simulink model "VCU_SW_2020"  (R2020b)
settings: Solver=FixedStepDiscrete  StartTime=0.0  StopTime=inf  FixedStep=1e-2  RelTol=1e-3
PreLoadFcn:
  | RTWConfigurationCB('preloadfcn', bdroot);
InitFcn:
  | loadvar_ttc500
undefined symbols (not defined in the file): BrkPedalTypes, CabMovModeTypes, cFuseTempSensAcc_X, cFuseTempSensAcc_Y, cFuseTempSensVal_X, cFuseTempSensVal_Y, cTMSTempSensVal_X, cTMSTempSensVal_Y, cTransferCaseSpeedRatio, diag_state, DoorsPositionTypes, dP_filter_Y, DriverOccClassSystemTypes, ErrorValueTypes, fatal_error_callback, IO_ADC_NO_RANGE, LadderStatusTypes, pAnalogCabRotSensAcc, pAnalogCabRotSensMaxVolt, pAnalogCabRotSensMinVolt, pAnalogCabRotSensRange, pAnalogCabRotSensZeroVolt, pBrkActivePress, pCabTiltSensAcc, pCabTiltSensMaxCur, pCabTiltSensMinCur, pDistanceCorrection, pECANManual_BPNEnable, pECANManual_BPNEnabler_Flag, pFilterSensAccRes, pHDirMaxDiffFrq, pHDirSensHighLvl, pHDirSensLowLvl, pMainGearRatio, pMaxFilterSensRes, pMaxFirstPedalSensValue, pMaxFuseTempSensRes, pMaxPressLoss, pMaxPressSensCurrent, pMaxPressValue, pMaxPressValueHydMotAndPump, pMaxPressValueParkDrain, pMaxSecondPedalSensValue, pMaxTempSensVoltage, pMaxTempValue, pMaxTMSTempSensRes, pMinFilterSensRes, pMinFirstPedalSensValue, pMinFuseTempSensRes, pMinPressLoss, pMinPressSensCurrent, pMinPressValue, pMinSecondPedalSensValue, pMinTempSensVoltage, pMinTempValue, pMinTMSTempSensRes, pMotorRingTeethNum, pPedalSensAccuracyPct, pPedalSensAccuracyVolt, pPressLossTreshhold ... (+20)
libraries: TTlibrary x270, canmsglib x127, simulink x88
(part 16 of 17)

== matlab function VCU_SW_2020/ServerFcn/convDIOStatusTypeToNum/MATLAB Function ==
  data: enum input; value output
function value = convertDIOStsToNumFcn(enum)
%#codegen
    if enum == StatusModeTypes.ON
        value = true;
    else
        value = false;
    end
% for future, if there is error or warning, then set function is not called
end

== matlab function VCU_SW_2020/InputLayer/InputInterfaces/AnalogInput/AIProc10msec/WasherTiltPumpTrans/getWasherTiltPumpTransSensDataFcn ==
  data: washerTiltPumpTransSens input; washerTiltPercent output; maxVolt input; minVolt input; accuracy input
function washerTiltPercent = getAnalogCabRotSensData(washerTiltPumpTransSens,...
     maxVolt, minVolt, accuracy)

 sensRange = single(maxVolt - minVolt)/single(2);
 zeroVolt = single(minVolt) + sensRange;
 
if (washerTiltPumpTransSens > (minVolt - accuracy)) &&...
   (washerTiltPumpTransSens < (maxVolt + accuracy)) %условие на попадание в диапазон датчика, при невыполнении - ошибка
    if washerTiltPumpTransSens > maxVolt %крайнее положение - остается
        washerTiltPercent = int8(100);
    elseif washerTiltPumpTransSens < minVolt %крайнее положение - остается
        washerTiltPercent = -int8(100);
    else
        if washerTiltPumpTransSens > zeroVolt
            helper = (single(washerTiltPumpTransSens) - single(zeroVolt))/single(sensRange)*single(100);
        elseif washerTiltPumpTransSens < zeroVolt 
            helper = -(single(zeroVolt) - single(washerTiltPumpTransSens))/single(sensRange)*single(100);
        else
            helper = single(0);
        end
        washerTiltPercent = int8(helper);
    end
else
   washerTiltPercent = int8(ErrorValueTypes.UNKNOWN_ERROR); 
end 
    
end

== matlab function VCU_SW_2020/InputLayer/InputInterfaces/DigitalInput/Function-Call Subsystem/MATLAB Function ==
  data: sensSupply1 input; sensSupply2 input
  events: fcncall output FUNCTION_CALL_EVENT
function fcn(sensSupply1, sensSupply2)

    persistent timer
        if isempty(timer)
            timer = uint8(0);
        end
        
    if sensSupply1 == StateModeTypes.STT_ENABLE && sensSupply2 == StateModeTypes.STT_ENABLE
        if timer < uint8(1000)
            timer = timer + uint8(1);
        end
    end
    
    if timer >= uint8(1000)
        fcncall();
    end
    
end

== matlab function VCU_SW_2020/InputLayer/InputInterfaces/DigitalInput/Function-Call Subsystem/cabRotIndSensProc/cabRotIndSensProc fcn ==
  data: pResetIndCabSensErr input
function cabRotIndSensProc(pResetIndCabSensErr)
    
    persistent err
    if isempty(err)
        err = false;
    end
    
    if err
        if pResetIndCabSensErr
            err = false;
            setIndSensErr(err);
        end        
    else
        cabRotPos = getIndRotSensData();
        if cabRotPos == CabRotPosTypes.ROTPOS_ERROR
            err = true;
            setIndSensErr(err);
        else
            setIndRotSensData(cabRotPos);
        end        
    end

end

== matlab function VCU_SW_2020/InputLayer/InputInterfaces/DigitalInput/Function-Call Subsystem/cabRotIndSensProc/getIndRotSensData/getIndRotSensData fcn ==
  data: indSensLeft input; cabPos output; indSensRight input
function cabPos = getIndRotSensData(indSensLeft, indSensRight)

    if (indSensRight == StateModeTypes.STT_ENABLE)&&...
       (indSensLeft == StateModeTypes.STT_ENABLE)
        cabPos = CabRotPosTypes.ROTPOS_NEAR_ZERO;
    elseif (indSensRight == StateModeTypes.STT_DISABLE)&&...
           (indSensLeft == StateModeTypes.STT_ENABLE)
        cabPos = CabRotPosTypes.ROTPOS_LEFT;
    elseif (indSensRight == StateModeTypes.STT_ENABLE)&&...
           (indSensLeft == StateModeTypes.STT_DISABLE)
        cabPos = CabRotPosTypes.ROTPOS_RIGHT;
    elseif (indSensRight == StateModeTypes.STT_DISABLE)&&...
           (indSensLeft == StateModeTypes.STT_DISABLE)
        switch getRotPos()
            case {CabRotPosTypes.ROTPOS_LEFT, CabRotPosTypes.ROTPOS_LEFT_END}
                cabPos = CabRotPosTypes.ROTPOS_LEFT_END;
            case {CabRotPosTypes.ROTPOS_RIGHT, CabRotPosTypes.ROTPOS_RIGHT_END}
                cabPos = CabRotPosTypes.ROTPOS_RIGHT_END;
            otherwise
                cabPos = CabRotPosTypes.ROTPOS_ERROR;
        end    
    else
        cabPos = CabRotPosTypes.ROTPOS_ERROR;
    end
    
end

== matlab function VCU_SW_2020/InputLayer/InputInterfaces/PWDInput/PWDProc100msec/MATLAB Function ==
  data: HMotorSpeed input; vehicleSpeed output; trCaseGear input; wheelRad input; finalDriveRatio input; lowRatio input; highRatio input; diagReplacement input; diagErrorValue input
function vehicleSpeed  = calculateVehicleSpeed(HMotorSpeed, trCaseGear,...
    wheelRad, finalDriveRatio, lowRatio, highRatio, ...
    diagReplacement, diagErrorValue)

if diagErrorValue ~= StateModeTypes.STT_ENABLE && ...
        diagReplacement ~= StateModeTypes.STT_ENABLE && ...
        HMotorSpeed ~= uint16(ErrorValueTypes.SPEED_ERROR_VALUE)
    if trCaseGear == GearNumTypes.GEAR_2_WHEEL_LOW || trCaseGear == GearNumTypes.GEAR_4_WHEEL_LOW
        vehicleSpeedRaw = single(HMotorSpeed)*wheelRad*60*2*pi/lowRatio/finalDriveRatio/1000;
        vehicleSpeed = uint8(vehicleSpeedRaw);
    elseif trCaseGear == GearNumTypes.GEAR_2_WHEEL_HIGH || trCaseGear == GearNumTypes.GEAR_4_WHEEL_HIGH
        vehicleSpeedRaw = single(HMotorSpeed)*wheelRad*60*2*pi/highRatio/finalDriveRatio/1000;
        vehicleSpeed = uint8(vehicleSpeedRaw);
   elseif trCaseGear == GearNumTypes.GEAR_NEUTRAL || trCaseGear == GearNumTypes.GEAR_NOT_AVAILABLE
        vehicleSpeed = uint8(0);    
    else
        vehicleSpeed = uint8(ErrorValueTypes.SPEED_ERROR_VALUE);
    end
else
    vehicleSpeed = uint8(ErrorValueTypes.SPEED_ERROR_VALUE);
end

== matlab function VCU_SW_2020/InputLayer/InputInterfaces/DigitalInput/Function-Call Subsystem1/MATLAB Function ==
  data: HighGear input; state output; LowGear input
function state = transCaseStt(HighGear, LowGear)

if HighGear == StateModeTypes.STT_DISABLE && LowGear == StateModeTypes.STT_DISABLE
    state = GearNumTypes.GEAR_NOT_AVAILABLE;
elseif ( HighGear == StateModeTypes.STT_ENABLE && ...
        LowGear == StateModeTypes.STT_DISABLE)
    state = GearNumTypes.GEAR_2_WHEEL_HIGH;
elseif ( HighGear == StateModeTypes.STT_DISABLE && ...
        LowGear == StateModeTypes.STT_ENABLE)
    state = GearNumTypes.GEAR_4_WHEEL_LOW;
else
    state = GearNumTypes.GEAR_ERROR;
end

end

== matlab function VCU_SW_2020/InputLayer/InputNetwork/InputCCAN/CCAN100msecProc1/InputTransSelect/calcLeverPos/MATLAB Function ==
  data: TransReqGear input; SelSig1 input; LeverPos output; SelSig2 input; SelSig3 input
function LeverPos = calculateLeverPosition(TransReqGear, SelSig1,...
    SelSig2, SelSig3)


if (TransReqGear == LeverPosTypes.NEUTRAL && SelSig1 == StateModeTypes.STT_ENABLE && ...
        SelSig2 ==StateModeTypes.STT_DISABLE && SelSig3 == StateModeTypes.STT_DISABLE)
    LeverPos = LeverPosTypes.NEUTRAL;
elseif (TransReqGear == LeverPosTypes.DRIVE && SelSig1 == StateModeTypes.STT_DISABLE && ...
        SelSig2 ==StateModeTypes.STT_ENABLE && SelSig3 == StateModeTypes.STT_DISABLE)
    LeverPos = LeverPosTypes.DRIVE;
elseif (TransReqGear == LeverPosTypes.REVERSE && SelSig1 == StateModeTypes.STT_DISABLE && ...
        SelSig2 ==StateModeTypes.STT_DISABLE && SelSig3 == StateModeTypes.STT_ENABLE)
    LeverPos = LeverPosTypes.REVERSE;
else
    if (SelSig1 == StateModeTypes.STT_ERROR || SelSig2 == StateModeTypes.STT_ERROR ||...
            SelSig3 == StateModeTypes.STT_ERROR)
        LeverPos = TransReqGear;
    elseif (TransReqGear == LeverPosTypes.LEVER_POS_ERROR || ...
            TransReqGear == LeverPosTypes.LEVER_POS_DOES_NOT_DEFINED)
        if (SelSig1 == StateModeTypes.STT_ENABLE && ...
                SelSig2 ==StateModeTypes.STT_DISABLE && SelSig3 == StateModeTypes.STT_DISABLE)
            LeverPos = LeverPosTypes.NEUTRAL;
        elseif (SelSig1 == StateModeTypes.STT_DISABLE && ...
                SelSig2 ==StateModeTypes.STT_ENABLE && SelSig3 == StateModeTypes.STT_DISABLE)
            LeverPos = LeverPosTypes.DRIVE;
        elseif (SelSig1 == StateModeTypes.STT_DISABLE && ...
                SelSig2 ==StateModeTypes.STT_DISABLE && SelSig3 == StateModeTypes.STT_ENABLE)
            LeverPos = LeverPosTypes.REVERSE;
        else
            LeverPos = LeverPosTypes.LEVER_POS_DOES_NOT_DEFINED;
        end
    else
        LeverPos = LeverPosTypes.LEVER_POS_DOES_NOT_DEFINED;
    end
end

== matlab function VCU_SW_2020/EEPROM Layer/calculate trip distance/calcTotalDistCtrl ==
  data: EEPROMData data_store_memory
  events: calcTotalDist output FUNCTION_CALL_EVENT
function calcTotalDistCtrl()
global EEPROMData

  if  EEPROMData.writingInProcessFl ~= StateModeTypes.STT_ENABLE
      calcTotalDist();
  end

end

== matlab function VCU_SW_2020/EEPROM Layer/calculate trip distance/EEPROM read1/calcTotalDist ==
  data: tripDist input; updDistM output; savedDistM input; savedDistKM input; savedDistKKM input; updDistKM output; updDistKKM output; updDistTotal output
function [updDistM, updDistKM, updDistKKM, updDistTotal] = calcTotalDist(tripDist, ...
    savedDistM, savedDistKM, savedDistKKM)

updDistTotal = tripDist ...
    + uint32(savedDistKKM) * uint32(1000000) ...
    + uint32(savedDistKM) * uint32(1000) ...
    + uint32(savedDistM);

if uint16((updDistTotal - uint32(500000)) / uint32(1000000)) < uint16(1000)
    updDistKKM = uint16((updDistTotal - uint32(500000)) / uint32(1000000));
else
   updDistKKM = uint16(0);
end

updDistKM = uint16((uint32(updDistTotal - uint32(updDistKKM) ...
    * uint32(1000000)) - uint32(500)) / uint32(1000));

updDistM = uint16(updDistTotal - uint32(updDistKKM) * ...
    uint32(1000000) - uint32(updDistKM) * uint32(1000));

end

== matlab function VCU_SW_2020/EEPROM Layer/updateUDSStruct/MATLAB Function ==
  data: EngineHours input; UDSStruct data_store_memory
function fcn(EngineHours)

    global UDSStruct
    
    persistent EngineHoursOnStartup
        if isempty(EngineHoursOnStartup)
            EngineHoursOnStartup = single(UDSStruct.TotalEngineHours)*single(20);
        end
        
    UDSStruct.TotalEngineHours = uint32(EngineHoursOnStartup + EngineHours*single(20));
    UDSStruct.CurEngineHours = uint32(EngineHours*single(20));
    
end

== matlab function VCU_SW_2020/EEPROM Layer/Simulink Function/eeprom_read_processing_kora ==
  data: UDSStruct data_store_memory; flag output; read_sts output
function [flag, read_sts] = readProcessing()

    global UDSStruct
    
    %Флаг успешной записи в структуру
    flag = false;
    
    eeprom_read_sts = uint16(15);
    
    if (coder.target('MATLAB')) || (coder.target('Sfun'))

    else
        %Получение флага успешного чтения из EEPROM
        read_flag = uint8(0);
        read_flag = coder.ceval('get_read_flag');
        
        %Получение даных после второго успешного чтения
        %Первое успешное чтение обман (с) Ваня
        if read_flag == 2

            data = zeros(10, 1, 'uint32');
            coder.ceval('get_EEPROM_data', data);
            eeprom_read_sts = coder.ceval('get_readSts');

            UDSStruct.DistanceM = uint16(data(1));
            UDSStruct.DistanceKM = uint16(data(2));
            UDSStruct.DistanceKKM = uint16(data(3));
            UDSStruct.EngineHours = uint32(data(4));
            UDSStruct.TransPumpVolumeMax = uint8(data(5));
            UDSStruct.TransMotorVolumeMin = uint8(data(6));
            UDSStruct.AccelerationPedalMaxEngSpd = uint8(data(7));
            UDSStruct.AccelerationPedalMinEngSpd = uint8(data(8));
            UDSStruct.EngineSpeedMax = uint16(data(9));
            UDSStruct.EngineSpeedMin = uint16(data(10));
            
            flag = true;
            
        end
        
    end
    
    read_sts = eeprom_read_sts;
    
end

== matlab function VCU_SW_2020/EEPROM Layer/EEPROM Client2 ==
  data: t15common input; sig1 input; sig2 input; read_flag output; write_flag output
function [read_flag, write_flag] = EEPROMControl(t15common, sig1, sig2)
    
    persistent data_read_successful data_write_successful t15common_old read_reqest write_reqest
        if isempty(data_read_successful)
            data_read_successful = false;
            data_write_successful = false;
            t15common_old = StateModeTypes.STT_DISABLE;
            read_reqest = false;
            write_reqest = false;
        end
        
    persistent sig1_old sig2_old
        if isempty(sig1_old)
            sig1_old = StateModeTypes.STT_DISABLE;
            sig2_old = StateModeTypes.STT_DISABLE;
        end
        
    if t15common_old == StateModeTypes.STT_DISABLE ...
       && t15common == StateModeTypes.STT_ENABLE
        read_reqest = true;
    elseif t15common_old == StateModeTypes.STT_ENABLE ...
           && t15common == StateModeTypes.STT_DISABLE 
        write_reqest = true;
        setDataToWrite();
    end
        
    if ~data_read_successful && read_reqest == true ...
       || sig1 == StateModeTypes.STT_ENABLE ...
          && sig1_old == StateModeTypes.STT_DISABLE
        data_read_successful = readProcessing();
    end
    
    if ~data_write_successful && write_reqest == true ...
       || sig2 == StateModeTypes.STT_ENABLE ...
          && sig2_old == StateModeTypes.STT_DISABLE
        data_write_successful = writeProcessing();
    end
    
    sig1_old = sig1;
    sig2_old = sig2;
    
    t15common_old = t15common;
    
    read_flag = data_read_successful;
    write_flag = data_write_successful;
    
    get_eeprom_status();
        
end
% global EEPROMData
% persistent cnt exT15state rst_cnt
% if isempty(cnt)
%     cnt = uint8(0);
%     exT15state = t15common;
%     rst_cnt = uint8(0);
% end
% 
% if EEPROMData.alreadyReadFlag ~= StateModeTypes.STT_ENABLE
%     readDistance();
% end
% 
% if t15common ~= StateModeTypes.STT_ENABLE && exT15state == StateModeTypes.STT_ENABLE
%     EEPROMData.writingInProcessFl = StateModeTypes.STT_ENABLE;
% end
% 
% if EEPROMData.writingInProcessFl == StateModeTypes.STT_ENABLE && cnt < uint8(50)
%     cnt = cnt + uint8(1);
% else
%     EEPROMData.writingInProcessFl = StateModeTypes.STT_DISABLE;
%     if cnt ~= uint8(0)
%         cnt = uint8(0);
%     end
% end
% 
% if EEPROMData.writingInProcessFl == StateModeTypes.STT_ENABLE
%     if cnt == uint8(15)
%         if EEPROMData.updatedDistM ~= EEPROMData.savedDistM
%             write();
%         end
%     end
% 
%     if cnt == uint8(48)
%          EEPROMData.tripDistM = uint32(0);
%     end
% end
% 
% if tripReset == uint8(1)
%     
%     if rst_cnt < uint8(200)
%         
%         rst_cnt = rst_cnt + uint8(1);
%         
%     else
%        
%         if EEPROMData.Trip_Reset ~= StateModeTypes.STT_ENABLE
%             
%             EEPROMData.Trip_Reset = StateModeTypes.STT_ENABLE;
%             
%         end
%         
%     end
%     
% else
%     
%     if rst_cnt > uint8(0)
%         
%         rst_cnt = uint8(0);
%         
%     end
%     
%     if EEPROMData.Trip_Reset ~= StateModeTypes.STT_DISABLE
%         
%         EEPROMData.Trip_Reset = StateModeTypes.STT_DISABLE;
%         
%     end
%     
% end
% 
% exT15state = t15common;

== matlab function VCU_SW_2020/InputLayer/InputInterfaces/PWDInput/PWDProc100msec/validatePedalSensValue/MATLAB Function ==
  data: firstSensValue input; SpdValue output; secondSensValue input
function SpdValue = validateSpdSensValues(firstSensValue, ...
    secondSensValue)
    if and(firstSensValue ~= uint16(ErrorValueTypes.SPEED_ERROR_VALUE), ...
            secondSensValue ~= uint16(ErrorValueTypes.SPEED_ERROR_VALUE))
            helper = (uint16(firstSensValue) + ...
                uint16(secondSensValue))/uint16(2);
            SpdValue = uint16(helper);
    else
        SpdValue = uint16(ErrorValueTypes.SPEED_ERROR_VALUE);
    end
end

== matlab function VCU_SW_2020/InputLayer/InputInterfaces/AnalogInput/AIProc1000msec/Filter/MATLAB Function1 ==
  data: maxRes input; filterState output; minRes input; sensorValue input; accuracyValue input; maxPress input; minPress input; Treshold input
function filterState = calculatePressureValue(maxRes, minRes, ...
    sensorValue, accuracyValue, maxPress, minPress, Treshold)

    if and((sensorValue > minRes - accuracyValue), ...
        (sensorValue < maxRes + accuracyValue))
        if sensorValue >= maxRes
            pressLoss = uint32(maxPress);
        elseif sensorValue <= minRes
            pressLoss = uint32(minPress);
        else
            sensRange = single(maxRes - minRes);
            pressRange = single(maxPress - minPress);
            helper = (single(sensorValue)-single(minRes))*pressRange/sensRange;
            pressLoss = uint32(helper);
        end
    else
        pressLoss = uint32(ErrorValueTypes.PRESSURE_ERROR_VALUE);
    end
    
    if pressLoss < Treshold
        filterState = StateModeTypes.STT_DISABLE;
    else
        filterState = StateModeTypes.STT_ENABLE;
    end
end

== matlab function VCU_SW_2020/InputLayer/InputInterfaces/AnalogInput/AIProc1000msec/TemperatureValues/calcCurPressSensVal/MATLAB Function1 ==
  data: maxValue input; temperature output; minValue input; sensorValue input; accuracyValue input; minTemp input; maxTemp input
function temperature = calculateTMSTemp(maxValue, minValue, ...
    sensorValue, accuracyValue, minTemp, maxTemp)
    %must add prohibition for incorrect accuracy value, check for max and
    %min values (max > min)
    if and((sensorValue > minValue - accuracyValue), ...
        (sensorValue > maxValue + accuracyValue))
        if sensorValue >= maxValue
            temperature = maxTemp;
        elseif sensorValue <= minValue
            temperature = minTemp;
        else
            sensRange = single(maxValue - minValue);
            tempRange = single(maxTemp - minTemp);
            helper = single(sensorValue - minValue)*tempRange/sensRange;
            helper = helper + single(minTemp);
            temperature = int16(helper);
        end
    else
        temperature = int16(ErrorValueTypes.TEMPERATURE_ERROR_VALUE);
    end
end

== matlab function VCU_SW_2020/InputLayer/InputInterfaces/AnalogInput/AIProc1000msec/TemperatureValues/calcTMSTemp/MATLAB Function ==
  data: maxValue input; temperature output; minValue input; sensorValue input; accuracyValue input; minTemp input; maxTemp input
function temperature = calculateTMSTemp(maxValue, minValue, ...
    sensorValue, accuracyValue, minTemp, maxTemp)
    %must add prohibition for incorrect accuracy value, check for max and
    %min values (max > min)
    if and((sensorValue > minValue - accuracyValue), ...
        (sensorValue > maxValue + accuracyValue))
        if sensorValue >= maxValue
            temperature = maxTemp;
        elseif sensorValue <= minValue
            temperature = minTemp;
        else
            sensRange = single(maxValue - minValue);
            tempRange = single(maxTemp - minTemp);
            helper = single(sensorValue - minValue)*tempRange/sensRange;
            helper = helper + single(minTemp);
            temperature = int16(helper);
        end
    else
        temperature = int16(ErrorValueTypes.TEMPERATURE_ERROR_VALUE);
    end
end

== matlab function VCU_SW_2020/OutputLayer/OutputNetwork/OutputCCAN/SetCCAN500msec/MATLAB Function6 ==
  data: input input; value output
function value = fcn(input)

if input == StateModeTypes.STT_DISABLE
    value = uint8(0);
elseif input == StateModeTypes.STT_ENABLE
    value = uint8(1);
else
    value = uint8(0);
end

== matlab function VCU_SW_2020/InputLayer/InputInterfaces/AnalogInput/AIProc1000msec/TemperatureValues/calcTMSTemp/customLookUpTableMF ==
  data: dataX input; valueOut output; dataY input; valueIn input
function valueOut = customLT(dataX, dataY, valueIn)

if length(dataX) == length(dataY)
    if valueIn <= dataX(1)
        valueOut = dataY(1);
    elseif valueIn >= dataX(length(dataX))
        valueOut = dataY(length(dataY));
    else

    end
else
    valueOut = single(0);
end
















end

== matlab function VCU_SW_2020/InputLayer/InputInterfaces/AnalogInput/AIProc100msec/PressureValues/calcCurPressSensVal/MATLAB Function ==
  data: maxValue input; pressureValue output; minValue input; sensorValue input; accuracyValue input; minPress input; maxPress input
function pressureValue = calculatePressureValue(maxValue, minValue, ...
    sensorValue, accuracyValue, minPress, maxPress)
    %must add prohibition for incorrect accuracy value, check for max and
    %min values (max > min)
    if and((sensorValue > minValue - accuracyValue), ...
        (sensorValue < maxValue + accuracyValue))
        if sensorValue >= maxValue
            pressureValue = maxPress;
        elseif sensorValue <= minValue
            pressureValue = minPress;
        else
            sensRange = single(maxValue - minValue);
            pressRange = single(maxPress - minPress);
            helper = (single(sensorValue)-single(minValue))*pressRange/sensRange;
            pressureValue = uint32(helper);
        end
    else
        pressureValue = uint32(ErrorValueTypes.PRESSURE_ERROR_VALUE);
    end
end

== matlab function VCU_SW_2020/InputLayer/InputInterfaces/AnalogInput/AIProc10msec/CabMovValues/Simulink Function/MATLAB Function1 ==
  data: cabTiltLongSens input; cabPitchAngle output; cabPitchAngleDir output
function [cabPitchAngle, cabPitchAngleDir] = cabPitchSensProc...
    (cabTiltLongSens)
    % ток в мкА
    
    if cabTiltLongSens > int16(0)
        cabPitchAngleDir = CabPitchDirTypes.PITCH_FORWARD;
        cabPitchAngle = uint16(abs(cabTiltLongSens));
    elseif cabTiltLongSens < int16(0)
        cabPitchAngleDir = CabPitchDirTypes.PITCH_BACKWARD;
        cabPitchAngle = uint16(abs(cabTiltLongSens));
    elseif cabTiltLongSens == int16(0)
        cabPitchAngleDir = CabPitchDirTypes.PITCH_STANDBY;
        cabPitchAngle = uint16(abs(cabTiltLongSens));
    else
        cabPitchAngleDir = CabPitchDirTypes.PITCH_NOT_DEFINED;
        cabPitchAngle = uint16(0);
    end
    
end

== matlab function VCU_SW_2020/InputLayer/InputInterfaces/AnalogInput/AIProc10msec/CabMovValues/Simulink Function1/MATLAB Function2 ==
  data: cabRollAngle output; cabRollAngleDir output; cabTiltTransSens input
function [cabRollAngle, cabRollAngleDir] = cabRollSensProc...
    (cabTiltTransSens)
    % ток в мкА
    
    if cabTiltTransSens > int16(0)
        cabRollAngleDir = CabRollDirTypes.ROLL_LEFT;
        cabRollAngle = uint16(abs(cabTiltTransSens));
    elseif cabTiltTransSens < int16(0)
        cabRollAngleDir = CabRollDirTypes.ROLL_RIGHT;
        cabRollAngle = uint16(abs(cabTiltTransSens));
    elseif cabTiltTransSens == int16(0)
        cabRollAngleDir = CabRollDirTypes.ROLL_STANDBY;
        cabRollAngle = uint16(abs(cabTiltTransSens));
    else
        cabRollAngleDir = CabRollDirTypes.ROLL_NOT_DEFINED;
        cabRollAngle = uint16(0);
    end
    
end

== matlab function VCU_SW_2020/InputLayer/InputInterfaces/AnalogInput/AIProc10msec/CabMovValues/cabRotAnalogSensProc fcn ==
  data: pResetAnalogCabRotSensErr input
function cabRotAnalogSensProc(pResetAnalogCabRotSensErr)
    
    persistent err
    if isempty(err)
        err = false;
    end
    
    if err
        if pResetAnalogCabRotSensErr
            err = false;
            setAnalogSensErr(err);
        end  
    else
        [cabAngleCh1, cabAngleCh2] = getAnalogCabRotSensData();
        if (cabAngleCh1 == int16(ErrorValueTypes.UNKNOWN_ERROR))||...
           (cabAngleCh2 == int16(ErrorValueTypes.UNKNOWN_ERROR))
            err = true;
            setAnalogSensErr(err);
        else
            setAnalogCabRotSensData(cabAngleCh1, cabAngleCh2);
        end        
    end
 
end

== matlab function VCU_SW_2020/InputLayer/InputInterfaces/AnalogInput/AIProc10msec/CabMovValues/cabTiltSensProc fcn ==
  data: pResetCabTiltSensErr input; pitchSens input; rollSens input
function cabTiltSensProc(pResetCabTiltSensErr, pitchSens, rollSens)
    
    persistent err
    if isempty(err)
        err = false;
    end
    
    if err 
        if pResetCabTiltSensErr
            err = false;
            setCabTiltSensErr(err);
        end    
    else
        [cabPitchAngle, cabRollAngle] = getSensData(pitchSens, rollSens);
        if (cabPitchAngle == int16(ErrorValueTypes.UNKNOWN_ERROR))||...
           (cabRollAngle == int16(ErrorValueTypes.UNKNOWN_ERROR))
            err = true;
            setCabTiltSensErr(err);
        else
            setCabTiltSensData(cabPitchAngle, cabRollAngle);
        end
    end
    
end

== matlab function VCU_SW_2020/InputLayer/InputInterfaces/AnalogInput/AIProc10msec/CabMovValues/frameTiltSensProc fcn ==
  data: pResetFrameTiltSensErr input; pitchSens input; rollSens input
function frameTiltSensProc(pResetFrameTiltSensErr, pitchSens, rollSens)
    
    persistent err
    if isempty(err)
        err = false;
    end
    
    if err
        if pResetFrameTiltSensErr
            err = false;
            setFrameTiltSensErr(err);
        end
    else
        [framePitchAngle, frameRollAngle] = getSensData(pitchSens, rollSens);
        if (frameRollAngle == int16(ErrorValueTypes.UNKNOWN_ERROR))||...
           (frameRollAngle == int16(ErrorValueTypes.UNKNOWN_ERROR))
            err = true;
            setFrameTiltSensErr(err);
        else
            setFrameTiltSensData(framePitchAngle, frameRollAngle);
        end
    end
    
end

== matlab function VCU_SW_2020/InputLayer/InputInterfaces/AnalogInput/AIProc10msec/CabMovValues/getAnalogCabRotSensData/getAnalogCabRotSensData fcn ==
  data: voltCh1 input; cabAngleCh1 output; voltCh2 input; sensRange input; maxVolt input; minVolt input; zeroVolt input; accuracy input; cabAngleCh2 output; transferRatio input
function [cabAngleCh1,cabAngleCh2] = getAnalogCabRotSensData(voltCh1,...
    voltCh2, sensRange, maxVolt, minVolt, zeroVolt, accuracy, transferRatio)
    
    cabAngleCh = zeros(2,1,'int16');
    voltCh = zeros(2,1,'uint16');
    voltCh(1) = voltCh1;
    voltCh(2) = voltCh2;
    
    if (maxVolt > minVolt)&&(minVolt - accuracy >= 0)
        for i = 1:2
            if (voltCh(i) > (minVolt - accuracy))&&(voltCh(i) < (maxVolt + accuracy))
                if voltCh(i) > maxVolt
                    cabAngleCh(i) = int16(single(sensRange)/single(transferRatio));
                elseif voltCh(i) < minVolt
                    cabAngleCh(i) = -int16(single(sensRange)/single(transferRatio));
                else
                    helper = single(sensRange)*((single(voltCh(i)) - single(zeroVolt))/(single(zeroVolt) - single(minVolt)))/single(transferRatio);
                    cabAngleCh(i) = int16(helper);
                end
            end
        end
        angleAcc = int16(single(sensRange)*(single(accuracy)/single(zeroVolt - minVolt))/single(transferRatio)); %+-
        if abs(cabAngleCh(1) + cabAngleCh(2)) < angleAcc*2
            cabAngleCh1 = cabAngleCh(1);
            cabAngleCh2 = cabAngleCh(2);
        else
            cabAngleCh1 = int16(ErrorValueTypes.UNKNOWN_ERROR);
            cabAngleCh2 = int16(ErrorValueTypes.UNKNOWN_ERROR);
        end
    else
        cabAngleCh1 = int16(ErrorValueTypes.UNKNOWN_ERROR);
        cabAngleCh2 = int16(ErrorValueTypes.UNKNOWN_ERROR);     
    end
    
end

== matlab function VCU_SW_2020/OutputLayer/OutputNetwork/OutputCCAN/SetCCAN100msec/MATLAB Function6 ==
  data: input input; value output
function value = fcn(input)

if input == StateModeTypes.STT_DISABLE
    value = uint8(0);
elseif input == StateModeTypes.STT_ENABLE
    value = uint8(1);
else
    value = uint8(0);
end

== matlab function VCU_SW_2020/InputLayer/InputInterfaces/AnalogInput/AIProc10msec/CabMovValues/getCabTiltSensData/Simulink Function/MATLAB Function5 ==
  data: cabTiltSens input; signedCabTiltAngle output; minCur input; maxCur input; accuracy input
function signedCabTiltAngle  = cabTiltSensProc...
    (cabTiltSens, minCur, maxCur, accuracy)
    % ток в мкА

    if (maxCur > minCur)&&(minCur - accuracy >= 0)
        if (cabTiltSens > minCur - accuracy)&&(cabTiltSens < maxCur + accuracy)
            if cabTiltSens > maxCur
                signedCabTiltAngle = int16(5400);
            elseif cabTiltSens < minCur
                signedCabTiltAngle = int16(-1)*int16(5400);
            else
                sens = single(cabTiltSens)/single(1000);
                sinus = (single(sens) - single(12))/single(8);
                signedCabTiltAngle = int16(asin(sinus)*single(10800)/single(pi));
            end
        else
            signedCabTiltAngle = int16(ErrorValueTypes.UNKNOWN_ERROR);
        end
    else
        signedCabTiltAngle = int16(ErrorValueTypes.UNKNOWN_ERROR);
    end
    
end

== matlab function VCU_SW_2020/InputLayer/InputInterfaces/AnalogInput/AIProc10msec/CabMovValues/setAnalogCabRotSensData/cabRotSensConv fcn ==
  data: cabAngleCh1 input; cabAngle output; cabAngleDir output; cabAngleCh2 input
function [cabAngle, cabAngleDir] = cabRotSensConv(cabAngleCh1,cabAngleCh2)
%Ch1 - CW Ch2 - CCW
    cabAngleRaw = single(cabAngleCh2 - cabAngleCh1)/2;
    if int16(cabAngleRaw) > int16(0)
        cabAngleDir = CabRotDirTypes.ROT_LEFT;
        cabAngle = uint16(abs(cabAngleRaw));
    elseif int16(cabAngleRaw) < int16(0)
        cabAngleDir = CabRotDirTypes.ROT_RIGHT;
        cabAngle = uint16(abs(cabAngleRaw));
    elseif int16(cabAngleRaw) == int16(0)
        cabAngleDir = CabRotDirTypes.ROT_STANDBY;
        cabAngle = uint16(abs(cabAngleRaw));
    else
        cabAngleDir = CabRotDirTypes.ROT_NOT_DEFINED;
        cabAngle = uint16(0);
    end
    
end

== matlab function VCU_SW_2020/InputLayer/InputInterfaces/AnalogInput/AIProc10msec/MATLAB Function ==
  events: fcncall output FUNCTION_CALL_EVENT
function fcn()

    persistent timer
        if isempty(timer)
            timer = uint8(0);
        end
    if timer < 200    
        timer = timer + uint8(1);
    else
        fcncall();
    end
    
end

== matlab function VCU_SW_2020/InputLayer/InputInterfaces/AnalogInput/AIProc10msec/PedalValues/MATLAB Function ==
  data: AccPedMode input; AccPedRamp input; AccPedLim input; AccPedPress input; Man_AccPedLvl output
function Man_AccPedLvl = fcn(AccPedMode, AccPedRamp, AccPedLim, AccPedPress)

persistent AccPedLvl
if isempty(AccPedLvl)
    AccPedLvl = single(0);
end

if and(AccPedMode == uint8(1), AccPedPress == uint8(1))
    if (AccPedLvl + AccPedRamp) < single(AccPedLim)
        AccPedLvl = AccPedLvl + AccPedRamp;
    else
        AccPedLvl = single(AccPedLim);
    end
else
    AccPedLvl = single(0);
end

Man_AccPedLvl = uint8(AccPedLvl);

end

== matlab function VCU_SW_2020/InputLayer/InputInterfaces/AnalogInput/AIProc10msec/PedalValues/calcPedalSensDirect/MATLAB Function ==
  data: maxValue input; pedalValue output; minValue input; sensorValue input; accuracyValue input
function pedalValue = calculatePedalValue(maxValue, minValue, sensorValue, accuracyValue)
%must add prohibition for incorrect accuracy value, check for max and
%min values (max > min)
if and((minValue - accuracyValue >= 0), (maxValue > minValue))
    if and((sensorValue > minValue - accuracyValue), ...
            (sensorValue < maxValue + accuracyValue))
        if sensorValue >= maxValue
            pedalValue = uint8(100);
        elseif sensorValue <= minValue
            pedalValue = uint8(0);
        else
            sensRange = maxValue - minValue;
            helper = single(sensorValue - minValue)/single(sensRange);
            helper = single(100)*helper;
            pedalValue = uint8(helper);
        end
    else
        pedalValue = uint8(ErrorValueTypes.PEDAL_ERROR_VALUE);
    end
else
    pedalValue = uint8(ErrorValueTypes.PEDAL_ERROR_VALUE);
end
end

== matlab function VCU_SW_2020/InputLayer/InputInterfaces/AnalogInput/AIProc10msec/PedalValues/validatePedalSensValue/MATLAB Function ==
  data: firstSensValue input; pedalValue output; secondSensValue input; accuracyValue input
function pedalValue = validatePedSensValues(firstSensValue, ...
    secondSensValue, accuracyValue)
    if and(firstSensValue ~= uint8(ErrorValueTypes.PEDAL_ERROR_VALUE), ...
            secondSensValue ~= uint8(ErrorValueTypes.PEDAL_ERROR_VALUE))
        diffValue = int16(firstSensValue) - int16(secondSensValue);
        diffValue = uint8(abs(diffValue));
        if diffValue <= accuracyValue
            helper = (uint16(firstSensValue) + ...
                uint16(secondSensValue))/uint16(2);
            pedalValue = uint8(helper);
        else
            pedalValue = uint8(ErrorValueTypes.PEDAL_ERROR_VALUE);
        end
    else
        pedalValue = uint8(ErrorValueTypes.PEDAL_ERROR_VALUE);
    end
end

== matlab function VCU_SW_2020/InputLayer/InputInterfaces/AnalogInput/AIProc10msec/PressureValues/Simulink Function/MATLAB Function ==
  data: pBrkActivePress input; stt output; pressFB input
function stt = brkPressFBproc(pBrkActivePress, pressFB)
    
    if pressFB ~= ErrorValueTypes.PRESSURE_ERROR_VALUE
        if pressFB >= pBrkActivePress
            stt = StateModeTypes.STT_ENABLE;
        else
            stt = StateModeTypes.STT_DISABLE;
        end
    else
        stt = StateModeTypes.STT_ERROR;
    end
    
end

== matlab function VCU_SW_2020/OutputLayer/OutputNetwork/OutputCCAN/SetCCAN1000msec/MATLAB Function6 ==
  data: input input; value output
function value = fcn(input)

if input == StateModeTypes.STT_DISABLE
    value = uint8(0);
elseif input == StateModeTypes.STT_ENABLE
    value = uint8(1);
else
    value = uint8(0);
end

== matlab function VCU_SW_2020/InputLayer/InputInterfaces/AnalogInput/AIProc10msec/PressureValues/calcCurPressSensVal/MATLAB Function ==
  data: maxValue input; pressureValue output; minValue input; sensorValue input; accuracyValue input; minPress input; maxPress input
function pressureValue = calculatePressureValue(maxValue, minValue, ...
    sensorValue, accuracyValue, minPress, maxPress)
    %must add prohibition for incorrect accuracy value, check for max and
    %min values (max > min)
    if and((sensorValue > (int32(minValue) - int32(accuracyValue))), ...
        (sensorValue < maxValue + accuracyValue))
        if sensorValue >= maxValue
            pressureValue = maxPress;
        elseif sensorValue <= minValue
            pressureValue = minPress;
        else
            sensRange = single(maxValue - minValue);
            pressRange = single(maxPress - minPress);
            helper = (single(sensorValue)-single(minValue))*pressRange/sensRange;
            pressureValue = uint32(helper);
        end
    else
        pressureValue = uint32(ErrorValueTypes.PRESSURE_ERROR_VALUE);
    end
end

== matlab function VCU_SW_2020/InputLayer/InputInterfaces/AnalogInput/AIProc10msec/PumpMotorDirections/calcRotDirSens/MATLAB Function ==
  data: HighLvl input; LowLvl input; RotDir output; sensorValue input; MaxDiffFrq input; SpdSensSig1 input; SpdSensSig2 input
function RotDir = calculateRotationDirection(HighLvl, LowLvl,...
    sensorValue, MaxDiffFrq, SpdSensSig1, SpdSensSig2)

if (sensorValue ~= uint16(ErrorValueTypes.VOLTAGE_ERROR_VALUE) && ...
        SpdSensSig1 ~= uint16(ErrorValueTypes.FREQ_ERROR_VALUE) && ...
        SpdSensSig2 ~= uint16(ErrorValueTypes.FREQ_ERROR_VALUE) && ...
        abs(SpdSensSig1-SpdSensSig2) <= MaxDiffFrq)
    if sensorValue >= HighLvl
        RotDir = HydroAgrRotDirTypes.H_ROT_CCW;
    elseif sensorValue <= LowLvl
        RotDir = HydroAgrRotDirTypes.H_ROT_CW;
    else
        RotDir = HydroAgrRotDirTypes.H_ROT_NOT_DEFINED;
    end
else
    RotDir = HydroAgrRotDirTypes.H_ROT_NOT_DEFINED;
end

== matlab function VCU_SW_2020/InputLayer/InputInterfaces/PWDInput/GetPWD100msec/MATLAB Function8 ==
  data: u input; y output; err input
function y = fcn(u,err)

% persistent y_prev
% 
% if isempty(y_prev)
%     
%     y_prev = uint32(0);
%     
% end

if err == uint16(0) && u >= uint32(40000)
    
    y = u;
    
% elseif err == uint16(101)
%     
%     y = y_prev;
    
else
    
    y = uint32(0);
    
end


end

== matlab function VCU_SW_2020/InputLayer/InputInterfaces/PWDInput/PWDProc100msec/MATLAB Function1 ==
  data: sig1 input; sig2 input; TeethNum input; out output
function out = fcn(sig1, sig2, TeethNum)

out = uint16((sig1+sig2)/(2*TeethNum));

== matlab function VCU_SW_2020/InputLayer/InputInterfaces/PWDInput/PWDProc100msec/MATLAB Function2 ==
  data: SensDist input; trCaseGear input; wheelRad input; finalDriveRatio input; lowRatio input; highRatio input; InputFunctionsData data_store_memory; T15 input; distance output
function distance = calculateVehicleSpeed(SensDist, trCaseGear,...
    wheelRad, finalDriveRatio, lowRatio, highRatio, T15)

persistent sum
if isempty(sum)
    sum = single(0);
end

if T15 == StateModeTypes.STT_ENABLE
    
    if trCaseGear == GearNumTypes.GEAR_2_WHEEL_LOW || trCaseGear == GearNumTypes.GEAR_4_WHEEL_LOW
        helper = single(SensDist)*wheelRad*2*pi/lowRatio/finalDriveRatio/1000;
    elseif trCaseGear == GearNumTypes.GEAR_2_WHEEL_HIGH || trCaseGear == GearNumTypes.GEAR_4_WHEEL_HIGH
        helper = single(SensDist)*wheelRad*2*pi/highRatio/finalDriveRatio/1000;
    else
        helper = single(0);
    end
    
    sum = single(sum) + single(helper);
    distance = single(sum);
else
    distance = single(sum);
end
end

== matlab function VCU_SW_2020/InputLayer/InputInterfaces/PWDInput/PWDProc100msec/calcSpdSens/MATLAB Function ==
  data: sensFreq input; Spd output; teethNum input
function Spd = SpdFcn(sensFreq, teethNum)
    
    if sensFreq ~= uint32(ErrorValueTypes.FREQ_ERROR_VALUE)
        shftSpdInit = single(sensFreq)*single(60)/single(teethNum);
        Spd = uint16(shftSpdInit);
    else
        Spd = uint16(ErrorValueTypes.SPEED_ERROR_VALUE);
    end
    
end

== matlab function VCU_SW_2020/InputLayer/InputInterfaces/PWMCurrentInput/PWMCur10msecProc/Simulink Function/MATLAB Function ==
  data: pValveActiveCur input; stt output; curFB input
function stt = brkCurFBproc(pValveActiveCur, curFB)
    
    if curFB ~= ErrorValueTypes.CURRENT_ERROR_VALUE
        if curFB >= pValveActiveCur
            stt = StateModeTypes.STT_ENABLE;
        else
            stt = StateModeTypes.STT_DISABLE;
        end
    else
        stt = StateModeTypes.STT_ERROR;
    end
    
end

== matlab function VCU_SW_2020/EEPROM Layer/updateUDSStruct/MATLAB Function1 ==
  data: Distance input; UDSStruct data_store_memory
function fcn(Distance)

    global UDSStruct
    
    persistent DistanceOnStartup
        if isempty(DistanceOnStartup)
            DistanceOnStartup = single(UDSStruct.TotalDistance)*single(8);
        end
        
    UDSStruct.TotalDistance = uint32(DistanceOnStartup + Distance*single(8));
    UDSStruct.CurDistance = uint32(Distance*single(8));
    
end

== matlab function VCU_SW_2020/InputLayer/InputNetwork/InputCCAN/GetCCAN100msec/CM3/MATLAB Function ==
  data: value input uint8; TransferCaseEnum output
function TransferCaseEnum = calcTrCaseGear(value)

    if value == uint8(0)
        TransferCaseEnum = GearNumTypes.GEAR_2_WHEEL_HIGH;
    elseif value == uint8(1) 
        TransferCaseEnum = GearNumTypes.GEAR_4_WHEEL_HIGH;
    elseif value == uint8(2) 
        TransferCaseEnum = GearNumTypes.GEAR_NEUTRAL;
    elseif value == uint8(3) 
        TransferCaseEnum = GearNumTypes.GEAR_2_WHEEL_LOW;
    elseif value == uint8(4) 
        TransferCaseEnum = GearNumTypes.GEAR_4_WHEEL_LOW;
    else
        TransferCaseEnum = GearNumTypes.GEAR_NOT_AVAILABLE;
    end
    
end

== matlab function VCU_SW_2020/InputLayer/InputNetwork/InputCCAN/GetCCAN1000msec/OCSI/MATLAB Function ==
  data: Value input; DriverOccClassSystem output
function DriverOccClassSystem = calcDriverOccClassSystem(Value)
    
    if Value == uint8(0)
        DriverOccClassSystem = DriverOccClassSystemTypes.DRIVER_CLASS_EMPTY;
    elseif Value > uint8(0) && Value < uint8(5)
        DriverOccClassSystem = DriverOccClassSystemTypes.DRIVER_CLASS_DRIVER_PRESENT;
    elseif Value == uint8(5)
        DriverOccClassSystem = DriverOccClassSystemTypes.DRIVER_CLASS_RESERVED;
    elseif Value == uint8(6)
        DriverOccClassSystem = DriverOccClassSystemTypes.DRIVER_CLASS_ERROR;
    else
        DriverOccClassSystem = DriverOccClassSystemTypes.DRIVER_CLASS_NOT_AVAILABLE;
    end
end

== matlab function VCU_SW_2020/InputLayer/InputNetwork/InputCCAN/GetCCAN100msec/Right Small Pan Cmd/MATLAB Function ==
  data: Value input; LadderStatus output
function LadderStatus = calcLadderStatus(Value)
    
    if Value == uint8(0)
        LadderStatus = LadderStatusTypes.LADDER_UP;
    elseif Value == uint8(1)
        LadderStatus = LadderStatusTypes.LADDER_DOWN;
    elseif Value == uint8(2)
        LadderStatus = LadderStatusTypes.LADDER_RESERVED;
    else
        LadderStatus = LadderStatusTypes.LADDER_NOT_AVAILABLE;
    end
end

== matlab function VCU_SW_2020/InputLayer/InputNetwork/InputCCAN/GetCCAN100msec/DC1/MATLAB Function ==
  data: Value input; PositionOfDoors output
function PositionOfDoors = calcPositionOfDoors(Value)
    
    if Value == uint8(0)
        PositionOfDoors = DoorsPositionTypes.DOORS_POS_AT_LEAST_1_DOOR_IS_OPEN;
    elseif Value == uint8(1)
        PositionOfDoors = DoorsPositionTypes.DOORS_POS_CLOSING_LAST_DOOR;
    elseif Value == uint8(2)
        PositionOfDoors = DoorsPositionTypes.DOORS_POS_ALL_DOORS_CLOSED;
    elseif Value > uint8(2) && Value < uint8(14)
        PositionOfDoors = DoorsPositionTypes.DOORS_POS_NOT_DEFINED;
    elseif Value == uint8(14)
        PositionOfDoors = DoorsPositionTypes.DOORS_POS_ERROR;
    else
        PositionOfDoors = DoorsPositionTypes.DOORS_POS_NOT_AVAILABLE;
    end
end

== matlab function VCU_SW_2020/InputLayer/InputNetwork/InputCCAN/GetCCAN100msec/TC1/MATLAB Function ==
  data: value input; leverPosEnum output
function leverPosEnum = calcLeverPosFcn(value)
        if value == uint16(hex2dec('DE'))
            leverPosEnum = LeverPosTypes.NEUTRAL;
        elseif value == uint16(hex2dec('FC'))
            leverPosEnum = LeverPosTypes.DRIVE;
        elseif value == uint16(hex2dec('DF'))
            leverPosEnum = LeverPosTypes.REVERSE;
        else
            leverPosEnum = LeverPosTypes.LEVER_POS_DOES_NOT_DEFINED;
        end
end

== matlab function VCU_SW_2020/InputLayer/InputNetwork/InputEngCAN/GetEngCAN1000msec/MATLAB Function ==
  data: Value input; coolLvlState output
function coolLvlState = convCoolLvl(Value)
if Value == uint8(0)
    coolLvlState = FluidStateTypes.FLUID_LEVEL_IS_CORRECT;
elseif Value == uint8(1)
    coolLvlState = FluidStateTypes.FLUID_LEVEL_IS_LOW;
else
    coolLvlState = FluidStateTypes.FLUID_STATE_IS_NOT_DEFINED;
end
end

== matlab function VCU_SW_2020/InputLayer/InputNetwork/InputEngCAN/GetEngCAN100msec/calcEnStrtM ==
  data: Value input; operatingMode output
function operatingMode = calcPperatingMode(Value)
    
    if Value == uint8(0)
        operatingMode = StarterModeTypes.START_NOT_REQ;
    elseif Value == uint8(1)
        operatingMode = StarterModeTypes.STARTER_ACT_GEAR_NOT_ENG;
    elseif Value == uint8(2)
        operatingMode = StarterModeTypes.STARTER_ACT_GEAR_ENG;
    elseif Value == uint8(3)
        operatingMode = StarterModeTypes.START_FINISHED;
    elseif Value == uint8(4)
        operatingMode = StarterModeTypes.STARTER_INH_ENG_RUN;
    elseif Value == uint8(5)
        operatingMode = StarterModeTypes.STARTER_INH_ENG_NOT_READY;
    elseif Value == uint8(6)
        operatingMode = StarterModeTypes.STARTER_INH_DRVL_ENG;
    elseif Value == uint8(7)
        operatingMode = StarterModeTypes.STARTER_INH_ACT_IMMO;
    elseif Value == uint8(8)
        operatingMode = StarterModeTypes.STARTER_INH_OVERHEAT;
    elseif Value == uint8(9)
        operatingMode = StarterModeTypes.START_RESERVED;
    elseif Value == uint8(10)
        operatingMode = StarterModeTypes.START_RESERVED;
    elseif Value == uint8(11)
        operatingMode = StarterModeTypes.START_RESERVED;
    elseif Value == uint8(12)
        operatingMode = StarterModeTypes.STARTER_INH_REASON_UNKNOWN;
    elseif Value == uint8(13)
        operatingMode = StarterModeTypes.START_ERROR;
    elseif Value == uint8(14)
        operatingMode = StarterModeTypes.START_ERROR;
    else
        operatingMode = StarterModeTypes.START_NOT_AVAILIBLE;
    end
end

== matlab function VCU_SW_2020/InputLayer/InputTimers/MATLAB Function ==
  data: u input; y output
  events: trigger input FUNCTION_CALL_EVENT
function y = fcn(u)

y = u;

== matlab function VCU_SW_2020/InputLayer/InputTimers/MATLAB Function1 ==
  data: u input; y output
  events: trigger input FUNCTION_CALL_EVENT
function y = fcn(u)

y = u;

== matlab function VCU_SW_2020/InputLayer/InputTimers/MATLAB Function2 ==
  data: u input; y output
  events: trigger input FUNCTION_CALL_EVENT
function y = fcn(u)

y = u;

== matlab function VCU_SW_2020/InputLayer/InputNetwork/InputStrCAN/Function-Call Subsystem/MATLAB Function1 ==
  data: neutralPos input; fwdPos input; bckwdPos input; absPos input; pos output; dir output
function [pos, dir] = fcn(neutralPos, fwdPos, bckwdPos, absPos)

    if absPos > single(100)
        pos = uint8(100);
    else
        pos = uint8(absPos);
    end

    if fwdPos == 1 &&...
       bckwdPos == 0
        dir = SteeringModeTypes.STEERING_RIGHT;
    elseif fwdPos == 0 &&...
           bckwdPos == 1
        dir = SteeringModeTypes.STEERING_LEFT;
    elseif neutralPos == 1
        dir = SteeringModeTypes.STEERING_HOLD;
    else
        dir = SteeringModeTypes.STEERING_NOT_AVAILABLE;
        pos = uint8(0);
    end

end

== matlab function VCU_SW_2020/InputLayer/Simulink Function1/MATLAB Function ==
  data: inpValue input; outValue output; errorSts input
function outValue = convCurValFcn(inpValue, errorSts)
%convert to mA if input data in μA!
if errorSts == uint16(0)
    outValue = inpValue;
    %outValue = uint16(inpValue);
else
    outValue = uint16(ErrorValueTypes.CURRENT_ERROR_VALUE);
end

end

== matlab function VCU_SW_2020/logSignal/daqFcn_mf ==
  data: diagTxEna input
  events: trigger input FUNCTION_CALL_EVENT
function daqFcn(diagTxEna)

    persistent i mode page 
    if isempty(i)
        i = uint8(1);
        mode = uint8(0);
        page = uint8(0);
    end

    [daqEna,pageNum,pageList,pageMode] = getDAQCmd();
    
    if daqEna == uint8(1) && diagTxEna == uint8(0)
        % pageMode
        % 0 - transmit all list of desired page
        % 1 - transmit only requested page of desired page
        if or(pageNum ~= page, pageMode ~= mode)
            i = uint8(1);
        end
        buffer = uint8(zeros(1,8));
        if pageMode == uint8(0)
            numList = getListNum(pageNum);
            if numList > uint8(0)
                [data,len] = getListData(pageNum,i);    
                if and(len > uint8(0),len < uint8(8))
                    buffer(1) = i;
                    for j = 1:length(data)
                        buffer(j+1) = data(j);
                    end
                    transmitDAQMsg(buffer);
                    i = i + uint8(1);
                    if i > numList
                        i = uint8(1);
                    end
                end 
            end        
        elseif pageMode == uint8(1)
            numList = getListNum(pageNum);
            if numList > uint8(0)
                [data,len] = getListData(pageNum,pageList);
                if and(len > uint8(0),len < uint8(8))
                    buffer(1) = pageList;
                    for j = 1:length(data)
                        buffer(j+1) = data(j);
                    end
                    transmitDAQMsg(buffer);
                end
            end
        end
    end
    mode = pageMode;
    page = pageNum;
end

== matlab function VCU_SW_2020/logSignal/getListData/Simulink Function/MATLAB Function ==
  data: value input; byte1 output; byte2 output
function [byte1, byte2] = fcn(value)

helper = bitand(value, uint16(255));
byte1 = uint8(helper);
helper = bitshift(value, -8);
helper = bitand(helper, uint16(255));
byte2 = uint8(helper);


end

== matlab function VCU_SW_2020/logSignal/getListData/Simulink Function1/MATLAB Function ==
  data: value input; byte1 output; byte2 output; byte3 output; byte4 output
function [byte1, byte2, byte3, byte4] = fcn(value)

helper = bitand(value, uint32(255));
byte1 = uint8(helper);
helper = bitshift(value, -8);
helper = bitand(helper, uint32(255));
byte2 = uint8(helper);
helper = bitshift(value, -16);
helper = bitand(helper, uint32(255));
byte3 = uint8(helper);
helper = bitshift(value, -24);
helper = bitand(helper, uint32(255));
byte4 = uint8(helper);

end
